simulink model "simulation_model"  (R2022a)
settings: Solver=VariableStepAuto  StartTime=0.0  StopTime=inf  FixedStep=0.02  MaxStep=0.1  RelTol=1e-3
values from neighbouring files (symbols this model uses):
  psi0 = atan(yc/xc)    [close_example.m]    (also in example_m.m)
  xc = coordinate(1)    [close_example.m]    (also in example_m.m)
  yc = coordinate(2)    [close_example.m]    (also in example_m.m)
undefined symbols (not defined in the file or in its folder): fuel_rate, gamma_pb, Pose, sigbuilder_block
libraries: simulink_extras x4, robotlib x3, simulink x1
(part 3 of 3)

== matlab function simulation_model/Parameters of rocket 9M723 and atmosphere model/Aerodynamic characteristics 9M723 ==
  data: Ma input; C_X0 output; C_Xa2 output; x_sm input; C_Na_kadl output; C_Na_ster output; x_sp output; C_ma output; C_mq output; x_sp_kadl output; x_sp_ster output
%% function which calculates Aerodynamic Force and Moment Coefficients
% 
% Inputs:
% Ma - number of Mach;
% x_sm - coordinate center of gravity [m]
%
% Outputs:
% C_X0 - Axial force coefficient (\alpha_t = 0)
% C_Xa2 - Derivative of axial force coefficient after sin^2\alpha_t
% C_Na_kadl - Derivative of normal force coefficient after sin\alpha for monocoque
% C_Na_ster - Derivative of normal force coefficient after sin\alpha for fins
% x_sp - coordinate center of pressure [m]
% C_ma - Derivative after pitch moment coefficient slope after sin\alpha
% C_mq - Pitch damping coefficient
% x_sp_kadl - coordinate center of pressure for monocoque [m]
% x_sp_ster - coordinate center of pressure for fins [m]


function [C_X0, C_Xa2, C_Na_kadl, C_Na_ster, x_sp, C_ma, C_mq, x_sp_kadl, x_sp_ster] = fcn(Ma, x_sm)

% Center of Gravity
CG = [2.8 3 3.3 3.5 3.7 4 4.4];

% Aerodynamic_Force_Coefficients
% [     Mach      CX0     CX2     CX4     CNa    CNa3    CPN     CYpa   CXfore  CXbase    CNq ]
AFC = [  0.01   0.216    2.81    3.12    3.92    3.12    3.92    0.00   0.000   0.068   0.148
         0.40   0.217    2.81    3.25    4.05    3.25    4.05    0.00   0.000   0.062   0.155
         0.60   0.217    2.81    3.31    4.12    3.31    4.12    0.00   0.000   0.058   0.158
         0.70   0.218    3.05    3.34    4.12    3.34    4.12    0.00   0.000   0.056   0.163
         0.75   0.219    3.17    3.35    4.12    3.35    4.12    0.00   0.000   0.054   0.165
         0.80   0.220    3.29    3.36    4.12    3.36    4.12    0.00   0.000   0.053   0.168
         0.85   0.232    3.53    3.41    4.15    3.41    4.15    0.00   0.000   0.062   0.170
         0.88   0.237    3.65    3.43    4.16    3.43    4.16    0.00   0.000   0.066   0.171
         0.90   0.243    3.76    3.45    4.17    3.45    4.17    0.00   0.000   0.071   0.172
         0.93   0.263    4.01    3.48    4.18    3.48    4.18    0.00   0.000   0.090   0.173
         0.95   0.283    4.25    3.50    4.18    3.50    4.18    0.00   0.000   0.108   0.174
         0.98   0.304    4.54    3.53    4.20    3.53    4.20    0.00   0.000   0.108   0.196
         1.00   0.325    4.83    3.56    4.22    3.56    4.22    0.00   0.000   0.108   0.217
         1.02   0.322    5.12    3.57    4.25    3.57    4.25    0.00   0.000   0.107   0.215
         1.05   0.319    5.41    3.58    4.28    3.58    4.28    0.00   0.000   0.105   0.214
         1.10   0.318    6.00    3.60    4.28    3.60    4.28    0.00   0.000   0.104   0.214
         1.20   0.310    6.65    3.62    4.23    3.62    4.23    0.00   0.000   0.100   0.210
         1.35   0.302    6.07    3.65    4.15    3.65    4.15    0.00   0.000   0.098   0.203
         1.50   0.288    5.46    3.71    4.04    3.71    4.04    0.00   0.000   0.092   0.196
         1.75   0.264    4.84    3.82    3.97    3.82    3.97    0.00   0.000   0.082   0.182
         2.00   0.245    4.24    3.81    3.89    3.81    3.89    0.00   0.000   0.078   0.167
         2.25   0.226    3.94    3.78    3.81    3.78    3.81    0.00   0.000   0.073   0.153
         2.50   0.206    3.63    3.75    3.74    3.75    3.74    0.00   0.000   0.068   0.138
         3.00   0.179    3.08    3.60    3.66    3.60    3.66    0.00   0.000   0.068   0.112
         3.50   0.163    2.82    3.46    3.56    3.46    3.56    0.00   0.000   0.070   0.093
         4.00   0.147    2.57    3.32    3.45    3.32    3.45    0.00   0.000   0.073   0.074
         4.50   0.137    2.32    3.24    3.41    3.24    3.41    0.00   0.000   0.075   0.062
         5.00   0.128    2.07    3.15    3.37    3.15    3.37    0.00   0.000   0.077   0.051
         6.00   0.114    1.85    3.08    3.32    3.08    3.32    0.00   0.000   0.078   0.037
         8.00   0.106    1.76    3.04    3.32    3.04    3.32    0.00   0.000   0.085   0.021];

%Aerodynamic Moment Coefficients for CG = 2800 mm
%          [ Mach     Cma     Cma3    Cma5    Cmq     Cmq2   Cnpa@1  Cnpa@3   Cnpa@5    Clp     Cld]
AMC_2800 = [  0.01   -2.75   -2.75  -135.7  -135.7   0.00   0.00   0.00   0.00   0.000  -0.501  0.0039
         0.40   -3.28   -3.28  -140.5  -140.5   0.00   0.00   0.00   0.00   0.000  -0.564  0.0045
         0.60   -3.56   -3.56  -143.0  -143.0   0.00   0.00   0.00   0.00   0.000  -0.596  0.0048
         0.70   -3.59   -3.59  -143.5  -143.5   0.00   0.00   0.00   0.00   0.000  -0.602  0.0048
         0.75   -3.61   -3.61  -143.8  -143.8   0.00   0.00   0.00   0.00   0.000  -0.605  0.0048
         0.80   -3.62   -3.62  -144.0  -144.0   0.00   0.00   0.00   0.00   0.000  -0.608  0.0049
         0.85   -3.75   -3.75  -146.6  -146.6   0.00   0.00   0.00   0.00   0.000  -0.624  0.0050
         0.88   -3.82   -3.82  -147.9  -147.9   0.00   0.00   0.00   0.00   0.000  -0.633  0.0051
         0.90   -3.89   -3.89  -149.2  -149.2   0.00   0.00   0.00   0.00   0.000  -0.641  0.0052
         0.93   -3.94   -3.94  -151.1  -151.1   0.00   0.00   0.00   0.00   0.000  -0.649  0.0052
         0.95   -3.99   -3.99  -153.0  -153.0   0.00   0.00   0.00   0.00   0.000  -0.657  0.0053
         0.98   -4.08   -4.08  -155.8  -155.8   0.00   0.00   0.00   0.00   0.000  -0.664  0.0054
         1.00   -4.17   -4.17  -158.6  -158.6   0.00   0.00   0.00   0.00   0.000  -0.670  0.0055
         1.02   -4.31   -4.31  -159.0  -159.0   0.00   0.00   0.00   0.00   0.000  -0.671  0.0055
         1.05   -4.45   -4.45  -159.4  -159.4   0.00   0.00   0.00   0.00   0.000  -0.671  0.0055
         1.10   -4.47   -4.47  -163.7  -163.7   0.00   0.00   0.00   0.00   0.000  -0.672  0.0055
         1.20   -4.29   -4.29  -165.6  -165.6   0.00   0.00   0.00   0.00   0.000  -0.651  0.0053
         1.35   -4.06   -4.06  -167.1  -167.1   0.00   0.00   0.00   0.00   0.000  -0.623  0.0051
         1.50   -3.69   -3.69  -168.6  -168.6   0.00   0.00   0.00   0.00   0.000  -0.596  0.0048
         1.75   -3.55   -3.55  -171.8  -171.8   0.00   0.00   0.00   0.00   0.000  -0.587  0.0048
         2.00   -3.21   -3.21  -171.4  -171.4   0.00   0.00   0.00   0.00   0.000  -0.531  0.0043
         2.25   -2.91   -2.91  -170.1  -170.1   0.00   0.00   0.00   0.00   0.000  -0.492  0.0040
         2.50   -2.61   -2.61  -168.7  -168.7   0.00   0.00   0.00   0.00   0.000  -0.452  0.0036
         3.00   -2.23   -2.23  -164.4  -164.4   0.00   0.00   0.00   0.00   0.000  -0.399  0.0032
         3.50   -1.79   -1.79  -158.7  -158.7   0.00   0.00   0.00   0.00   0.000  -0.353  0.0028
         4.00   -1.35   -1.35  -153.0  -153.0   0.00   0.00   0.00   0.00   0.000  -0.307  0.0024
         4.50   -1.19   -1.19  -148.9  -148.9   0.00   0.00   0.00   0.00   0.000  -0.291  0.0022
         5.00   -1.02   -1.02  -144.7  -144.7   0.00   0.00   0.00   0.00   0.000  -0.275  0.0021
         6.00   -0.87   -0.87  -141.6  -141.6   0.00   0.00   0.00   0.00   0.000  -0.261  0.0020
         8.00   -0.83   -0.83  -140.4  -140.4   0.00   0.00   0.00   0.00   0.000  -0.257  0.0019];

%Aerodynamic Moment Coefficients for CG = 3000 mm
%          [ Mach     Cma     Cma3    Cma5    Cmq     Cmq2   Cnpa@1  Cnpa@3   Cnpa@5    Clp     Cld]
AMC_3000 = [0.01   -2.07   -2.07  -124.4  -124.4   0.00   0.00   0.00   0.00   0.000  -0.501  0.0039
         0.40   -2.58   -2.58  -128.8  -128.8   0.00   0.00   0.00   0.00   0.000  -0.564  0.0045
         0.60   -2.84   -2.84  -131.1  -131.1   0.00   0.00   0.00   0.00   0.000  -0.596  0.0048
         0.70   -2.87   -2.87  -131.5  -131.5   0.00   0.00   0.00   0.00   0.000  -0.602  0.0048
         0.75   -2.88   -2.88  -131.7  -131.7   0.00   0.00   0.00   0.00   0.000  -0.605  0.0048
         0.80   -2.89   -2.89  -132.0  -132.0   0.00   0.00   0.00   0.00   0.000  -0.608  0.0049
         0.85   -3.01   -3.01  -134.5  -134.5   0.00   0.00   0.00   0.00   0.000  -0.624  0.0050
         0.88   -3.08   -3.08  -135.8  -135.8   0.00   0.00   0.00   0.00   0.000  -0.633  0.0051
         0.90   -3.14   -3.14  -137.1  -137.1   0.00   0.00   0.00   0.00   0.000  -0.641  0.0052
         0.93   -3.18   -3.18  -138.9  -138.9   0.00   0.00   0.00   0.00   0.000  -0.649  0.0052
         0.95   -3.23   -3.23  -140.7  -140.7   0.00   0.00   0.00   0.00   0.000  -0.657  0.0053
         0.98   -3.32   -3.32  -143.5  -143.5   0.00   0.00   0.00   0.00   0.000  -0.664  0.0054
         1.00   -3.40   -3.40  -146.2  -146.2   0.00   0.00   0.00   0.00   0.000  -0.670  0.0055
         1.02   -3.53   -3.53  -146.6  -146.6   0.00   0.00   0.00   0.00   0.000  -0.671  0.0055
         1.05   -3.67   -3.67  -147.0  -147.0   0.00   0.00   0.00   0.00   0.000  -0.671  0.0055
         1.10   -3.68   -3.68  -151.4  -151.4   0.00   0.00   0.00   0.00   0.000  -0.672  0.0055
         1.20   -3.51   -3.51  -153.6  -153.6   0.00   0.00   0.00   0.00   0.000  -0.651  0.0053
         1.35   -3.26   -3.26  -155.8  -155.8   0.00   0.00   0.00   0.00   0.000  -0.623  0.0051
         1.50   -2.88   -2.88  -158.5  -158.5   0.00   0.00   0.00   0.00   0.000  -0.596  0.0048
         1.75   -2.72   -2.72  -161.8  -161.8   0.00   0.00   0.00   0.00   0.000  -0.587  0.0048
         2.00   -2.38   -2.38  -161.7  -161.7   0.00   0.00   0.00   0.00   0.000  -0.531  0.0043
         2.25   -2.08   -2.08  -160.7  -160.7   0.00   0.00   0.00   0.00   0.000  -0.492  0.0040
         2.50   -1.79   -1.79  -159.7  -159.7   0.00   0.00   0.00   0.00   0.000  -0.452  0.0036
         3.00   -1.45   -1.45  -155.8  -155.8   0.00   0.00   0.00   0.00   0.000  -0.399  0.0032
         3.50   -1.04   -1.04  -150.5  -150.5   0.00   0.00   0.00   0.00   0.000  -0.353  0.0028
         4.00   -0.63   -0.63  -145.1  -145.1   0.00   0.00   0.00   0.00   0.000  -0.307  0.0024
         4.50   -0.48   -0.48  -141.1  -141.1   0.00   0.00   0.00   0.00   0.000  -0.291  0.0022
         5.00   -0.33   -0.33  -137.0  -137.0   0.00   0.00   0.00   0.00   0.000  -0.275  0.0021
         6.00   -0.20   -0.20  -134.1  -134.1   0.00   0.00   0.00   0.00   0.000  -0.261  0.0020
         8.00   -0.17   -0.17  -132.9  -132.9   0.00   0.00   0.00   0.00   0.000  -0.257  0.0019];

%Aerodynamic Moment Coefficients for CG = 3300 mm
%         [ Mach     Cma     Cma3    Cma5    Cmq     Cmq2   Cnpa@1  Cnpa@3   Cnpa@5    Clp     Cld]
AMC_3300 = [0.01   -1.05   -1.05  -107.9  -107.9   0.00   0.00   0.00   0.00   0.000  -0.501  0.0039
         0.40   -1.52   -1.52  -111.6  -111.6   0.00   0.00   0.00   0.00   0.000  -0.564  0.0045
         0.60   -1.76   -1.76  -113.5  -113.5   0.00   0.00   0.00   0.00   0.000  -0.596  0.0048
         0.70   -1.78   -1.78  -113.9  -113.9   0.00   0.00   0.00   0.00   0.000  -0.602  0.0048
         0.75   -1.79   -1.79  -114.1  -114.1   0.00   0.00   0.00   0.00   0.000  -0.605  0.0048
         0.80   -1.80   -1.80  -114.3  -114.3   0.00   0.00   0.00   0.00   0.000  -0.608  0.0049
         0.85   -1.90   -1.90  -116.8  -116.8   0.00   0.00   0.00   0.00   0.000  -0.624  0.0050
         0.88   -1.96   -1.96  -118.0  -118.0   0.00   0.00   0.00   0.00   0.000  -0.633  0.0051
         0.90   -2.01   -2.01  -119.2  -119.2   0.00   0.00   0.00   0.00   0.000  -0.641  0.0052
         0.93   -2.05   -2.05  -121.0  -121.0   0.00   0.00   0.00   0.00   0.000  -0.649  0.0052
         0.95   -2.09   -2.09  -122.7  -122.7   0.00   0.00   0.00   0.00   0.000  -0.657  0.0053
         0.98   -2.16   -2.16  -125.4  -125.4   0.00   0.00   0.00   0.00   0.000  -0.664  0.0054
         1.00   -2.24   -2.24  -128.0  -128.0   0.00   0.00   0.00   0.00   0.000  -0.670  0.0055
         1.02   -2.37   -2.37  -128.4  -128.4   0.00   0.00   0.00   0.00   0.000  -0.671  0.0055
         1.05   -2.50   -2.50  -128.8  -128.8   0.00   0.00   0.00   0.00   0.000  -0.671  0.0055
         1.10   -2.51   -2.51  -133.3  -133.3   0.00   0.00   0.00   0.00   0.000  -0.672  0.0055
         1.20   -2.33   -2.33  -135.9  -135.9   0.00   0.00   0.00   0.00   0.000  -0.651  0.0053
         1.35   -2.07   -2.07  -139.2  -139.2   0.00   0.00   0.00   0.00   0.000  -0.623  0.0051
         1.50   -1.67   -1.67  -143.8  -143.8   0.00   0.00   0.00   0.00   0.000  -0.596  0.0048
         1.75   -1.47   -1.47  -147.1  -147.1   0.00   0.00   0.00   0.00   0.000  -0.587  0.0048
         2.00   -1.14   -1.14  -147.6  -147.6   0.00   0.00   0.00   0.00   0.000  -0.531  0.0043
         2.25   -0.85   -0.85  -147.0  -147.0   0.00   0.00   0.00   0.00   0.000  -0.492  0.0040
         2.50   -0.57   -0.57  -146.5  -146.5   0.00   0.00   0.00   0.00   0.000  -0.452  0.0036
         3.00   -0.27   -0.27  -143.1  -143.1   0.00   0.00   0.00   0.00   0.000  -0.399  0.0032
         3.50    0.09    0.09  -138.3  -138.3   0.00   0.00   0.00   0.00   0.000  -0.353  0.0028
         4.00    0.45    0.45  -133.4  -133.4   0.00   0.00   0.00   0.00   0.000  -0.307  0.0024
         4.50    0.57    0.57  -129.5  -129.5   0.00   0.00   0.00   0.00   0.000  -0.291  0.0022
         5.00    0.69    0.69  -125.6  -125.6   0.00   0.00   0.00   0.00   0.000  -0.275  0.0021
         6.00    0.81    0.81  -122.9  -122.9   0.00   0.00   0.00   0.00   0.000  -0.261  0.0020
         8.00    0.83    0.83  -121.7  -121.7   0.00   0.00   0.00   0.00   0.000  -0.257  0.0019];

%Aerodynamic Moment Coefficients for CG = 3500 mm
%         [ Mach     Cma     Cma3    Cma5    Cmq     Cmq2   Cnpa@1  Cnpa@3   Cnpa@5    Clp     Cld]
AMC_3500 = [0.01   -0.37   -0.37   -97.1   -97.1   0.00   0.00   0.00   0.00   0.000  -0.501  0.0039
         0.40   -0.81   -0.81  -100.4  -100.4   0.00   0.00   0.00   0.00   0.000  -0.564  0.0045
         0.60   -1.04   -1.04  -102.1  -102.1   0.00   0.00   0.00   0.00   0.000  -0.596  0.0048
         0.70   -1.05   -1.05  -102.4  -102.4   0.00   0.00   0.00   0.00   0.000  -0.602  0.0048
         0.75   -1.06   -1.06  -102.6  -102.6   0.00   0.00   0.00   0.00   0.000  -0.605  0.0048
         0.80   -1.07   -1.07  -102.8  -102.8   0.00   0.00   0.00   0.00   0.000  -0.608  0.0049
         0.85   -1.16   -1.16  -105.2  -105.2   0.00   0.00   0.00   0.00   0.000  -0.624  0.0050
         0.88   -1.21   -1.21  -106.4  -106.4   0.00   0.00   0.00   0.00   0.000  -0.633  0.0051
         0.90   -1.26   -1.26  -107.6  -107.6   0.00   0.00   0.00   0.00   0.000  -0.641  0.0052
         0.93   -1.30   -1.30  -109.3  -109.3   0.00   0.00   0.00   0.00   0.000  -0.649  0.0052
         0.95   -1.33   -1.33  -111.0  -111.0   0.00   0.00   0.00   0.00   0.000  -0.657  0.0053
         0.98   -1.40   -1.40  -113.6  -113.6   0.00   0.00   0.00   0.00   0.000  -0.664  0.0054
         1.00   -1.46   -1.46  -116.2  -116.2   0.00   0.00   0.00   0.00   0.000  -0.670  0.0055
         1.02   -1.59   -1.59  -116.6  -116.6   0.00   0.00   0.00   0.00   0.000  -0.671  0.0055
         1.05   -1.72   -1.72  -117.0  -117.0   0.00   0.00   0.00   0.00   0.000  -0.671  0.0055
         1.10   -1.73   -1.73  -121.5  -121.5   0.00   0.00   0.00   0.00   0.000  -0.672  0.0055
         1.20   -1.54   -1.54  -124.5  -124.5   0.00   0.00   0.00   0.00   0.000  -0.651  0.0053
         1.35   -1.28   -1.28  -128.5  -128.5   0.00   0.00   0.00   0.00   0.000  -0.623  0.0051
         1.50   -0.86   -0.86  -134.2  -134.2   0.00   0.00   0.00   0.00   0.000  -0.596  0.0048
         1.75   -0.64   -0.64  -137.6  -137.6   0.00   0.00   0.00   0.00   0.000  -0.587  0.0048
         2.00   -0.31   -0.31  -138.5  -138.5   0.00   0.00   0.00   0.00   0.000  -0.531  0.0043
         2.25   -0.03   -0.03  -138.1  -138.1   0.00   0.00   0.00   0.00   0.000  -0.492  0.0040
         2.50    0.25    0.25  -137.8  -137.8   0.00   0.00   0.00   0.00   0.000  -0.452  0.0036
         3.00    0.51    0.51  -134.8  -134.8   0.00   0.00   0.00   0.00   0.000  -0.399  0.0032
         3.50    0.84    0.84  -130.3  -130.3   0.00   0.00   0.00   0.00   0.000  -0.353  0.0028
         4.00    1.17    1.17  -125.8  -125.8   0.00   0.00   0.00   0.00   0.000  -0.307  0.0024
         4.50    1.28    1.28  -122.0  -122.0   0.00   0.00   0.00   0.00   0.000  -0.291  0.0022
         5.00    1.38    1.38  -118.2  -118.2   0.00   0.00   0.00   0.00   0.000  -0.275  0.0021
         6.00    1.48    1.48  -115.5  -115.5   0.00   0.00   0.00   0.00   0.000  -0.261  0.0020
         8.00    1.49    1.49  -114.4  -114.4   0.00   0.00   0.00   0.00   0.000  -0.257  0.0019];

%Aerodynamic Moment Coefficients for CG = 3700 mm
%          [ Mach     Cma     Cma3    Cma5    Cmq     Cmq2   Cnpa@1  Cnpa@3   Cnpa@5    Clp     Cld]
AMC_3700 = [0.01    0.31    0.31   -86.4   -86.4   0.00   0.00   0.00   0.00   0.000  -0.501  0.0039
         0.40   -0.11   -0.11   -89.4   -89.4   0.00   0.00   0.00   0.00   0.000  -0.564  0.0045
         0.60   -0.32   -0.32   -90.9   -90.9   0.00   0.00   0.00   0.00   0.000  -0.596  0.0048
         0.70   -0.33   -0.33   -91.2   -91.2   0.00   0.00   0.00   0.00   0.000  -0.602  0.0048
         0.75   -0.33   -0.33   -91.3   -91.3   0.00   0.00   0.00   0.00   0.000  -0.605  0.0048
         0.80   -0.34   -0.34   -91.5   -91.5   0.00   0.00   0.00   0.00   0.000  -0.608  0.0049
         0.85   -0.42   -0.42   -93.8   -93.8   0.00   0.00   0.00   0.00   0.000  -0.624  0.0050
         0.88   -0.47   -0.47   -95.0   -95.0   0.00   0.00   0.00   0.00   0.000  -0.633  0.0051
         0.90   -0.51   -0.51   -96.2   -96.2   0.00   0.00   0.00   0.00   0.000  -0.641  0.0052
         0.93   -0.54   -0.54   -97.9   -97.9   0.00   0.00   0.00   0.00   0.000  -0.649  0.0052
         0.95   -0.57   -0.57   -99.5   -99.5   0.00   0.00   0.00   0.00   0.000  -0.657  0.0053
         0.98   -0.63   -0.63  -102.1  -102.1   0.00   0.00   0.00   0.00   0.000  -0.664  0.0054
         1.00   -0.69   -0.69  -104.7  -104.7   0.00   0.00   0.00   0.00   0.000  -0.670  0.0055
         1.02   -0.82   -0.82  -105.1  -105.1   0.00   0.00   0.00   0.00   0.000  -0.671  0.0055
         1.05   -0.94   -0.94  -105.4  -105.4   0.00   0.00   0.00   0.00   0.000  -0.671  0.0055
         1.10   -0.94   -0.94  -109.9  -109.9   0.00   0.00   0.00   0.00   0.000  -0.672  0.0055
         1.20   -0.75   -0.75  -113.2  -113.2   0.00   0.00   0.00   0.00   0.000  -0.651  0.0053
         1.35   -0.48   -0.48  -118.0  -118.0   0.00   0.00   0.00   0.00   0.000  -0.623  0.0051
         1.50   -0.06   -0.06  -124.8  -124.8   0.00   0.00   0.00   0.00   0.000  -0.596  0.0048
         1.75    0.19    0.19  -128.3  -128.3   0.00   0.00   0.00   0.00   0.000  -0.587  0.0048
         2.00    0.52    0.52  -129.5  -129.5   0.00   0.00   0.00   0.00   0.000  -0.531  0.0043
         2.25    0.79    0.79  -129.4  -129.4   0.00   0.00   0.00   0.00   0.000  -0.492  0.0040
         2.50    1.07    1.07  -129.3  -129.3   0.00   0.00   0.00   0.00   0.000  -0.452  0.0036
         3.00    1.29    1.29  -126.7  -126.7   0.00   0.00   0.00   0.00   0.000  -0.399  0.0032
         3.50    1.60    1.60  -122.4  -122.4   0.00   0.00   0.00   0.00   0.000  -0.353  0.0028
         4.00    1.89    1.89  -118.2  -118.2   0.00   0.00   0.00   0.00   0.000  -0.307  0.0024
         4.50    1.98    1.98  -114.5  -114.5   0.00   0.00   0.00   0.00   0.000  -0.291  0.0022
         5.00    2.07    2.07  -110.8  -110.8   0.00   0.00   0.00   0.00   0.000  -0.275  0.0021
         6.00    2.14    2.14  -108.2  -108.2   0.00   0.00   0.00   0.00   0.000  -0.261  0.0020
         8.00    2.15    2.15  -107.1  -107.1   0.00   0.00   0.00   0.00   0.000  -0.257  0.0019];

%Aerodynamic Moment Coefficients for CG = 4000 mm
%         [ Mach     Cma     Cma3    Cma5    Cmq     Cmq2   Cnpa@1  Cnpa@3   Cnpa@5    Clp     Cld]
AMC_4000 = [0.01    1.32    1.32   -70.8   -70.8   0.00   0.00   0.00   0.00   0.000  -0.501  0.0039
         0.40    0.95    0.95   -73.2   -73.2   0.00   0.00   0.00   0.00   0.000  -0.564  0.0045
         0.60    0.76    0.76   -74.4   -74.4   0.00   0.00   0.00   0.00   0.000  -0.596  0.0048
         0.70    0.76    0.76   -74.7   -74.7   0.00   0.00   0.00   0.00   0.000  -0.602  0.0048
         0.75    0.76    0.76   -74.8   -74.8   0.00   0.00   0.00   0.00   0.000  -0.605  0.0048
         0.80    0.76    0.76   -74.9   -74.9   0.00   0.00   0.00   0.00   0.000  -0.608  0.0049
         0.85    0.69    0.69   -77.2   -77.2   0.00   0.00   0.00   0.00   0.000  -0.624  0.0050
         0.88    0.65    0.65   -78.3   -78.3   0.00   0.00   0.00   0.00   0.000  -0.633  0.0051
         0.90    0.61    0.61   -79.5   -79.5   0.00   0.00   0.00   0.00   0.000  -0.641  0.0052
         0.93    0.59    0.59   -81.1   -81.1   0.00   0.00   0.00   0.00   0.000  -0.649  0.0052
         0.95    0.57    0.57   -82.8   -82.8   0.00   0.00   0.00   0.00   0.000  -0.657  0.0053
         0.98    0.52    0.52   -85.3   -85.3   0.00   0.00   0.00   0.00   0.000  -0.664  0.0054
         1.00    0.47    0.47   -87.8   -87.8   0.00   0.00   0.00   0.00   0.000  -0.670  0.0055
         1.02    0.35    0.35   -88.1   -88.1   0.00   0.00   0.00   0.00   0.000  -0.671  0.0055
         1.05    0.23    0.23   -88.5   -88.5   0.00   0.00   0.00   0.00   0.000  -0.671  0.0055
         1.10    0.23    0.23   -93.1   -93.1   0.00   0.00   0.00   0.00   0.000  -0.672  0.0055
         1.20    0.43    0.43   -96.8   -96.8   0.00   0.00   0.00   0.00   0.000  -0.651  0.0053
         1.35    0.71    0.71  -102.6  -102.6   0.00   0.00   0.00   0.00   0.000  -0.623  0.0051
         1.50    1.15    1.15  -111.2  -111.2   0.00   0.00   0.00   0.00   0.000  -0.596  0.0048
         1.75    1.43    1.43  -114.7  -114.7   0.00   0.00   0.00   0.00   0.000  -0.587  0.0048
         2.00    1.76    1.76  -116.4  -116.4   0.00   0.00   0.00   0.00   0.000  -0.531  0.0043
         2.25    2.03    2.03  -116.6  -116.6   0.00   0.00   0.00   0.00   0.000  -0.492  0.0040
         2.50    2.29    2.29  -116.9  -116.9   0.00   0.00   0.00   0.00   0.000  -0.452  0.0036
         3.00    2.47    2.47  -114.7  -114.7   0.00   0.00   0.00   0.00   0.000  -0.399  0.0032
         3.50    2.72    2.72  -110.9  -110.9   0.00   0.00   0.00   0.00   0.000  -0.353  0.0028
         4.00    2.98    2.98  -107.0  -107.0   0.00   0.00   0.00   0.00   0.000  -0.307  0.0024
         4.50    3.04    3.04  -103.5  -103.5   0.00   0.00   0.00   0.00   0.000  -0.291  0.0022
         5.00    3.09    3.09  -100.0  -100.0   0.00   0.00   0.00   0.00   0.000  -0.275  0.0021
         6.00    3.15    3.15   -97.5   -97.5   0.00   0.00   0.00   0.00   0.000  -0.261  0.0020
         8.00    3.14    3.14   -96.4   -96.4   0.00   0.00   0.00   0.00   0.000  -0.257  0.0019];

%Aerodynamic Moment Coefficients for CG = 4400 mm
%          [ Mach     Cma     Cma3    Cma5    Cmq     Cmq2   Cnpa@1  Cnpa@3   Cnpa@5    Clp     Cld]
AMC_4400 = [0.01    2.68    2.68   -50.5   -50.5   0.00   0.00   0.00   0.00   0.000  -0.501  0.0039
         0.40    2.36    2.36   -52.3   -52.3   0.00   0.00   0.00   0.00   0.000  -0.564  0.0045
         0.60    2.20    2.20   -53.2   -53.2   0.00   0.00   0.00   0.00   0.000  -0.596  0.0048
         0.70    2.21    2.21   -53.4   -53.4   0.00   0.00   0.00   0.00   0.000  -0.602  0.0048
         0.75    2.22    2.22   -53.5   -53.5   0.00   0.00   0.00   0.00   0.000  -0.605  0.0048
         0.80    2.22    2.22   -53.6   -53.6   0.00   0.00   0.00   0.00   0.000  -0.608  0.0049
         0.85    2.17    2.17   -55.8   -55.8   0.00   0.00   0.00   0.00   0.000  -0.624  0.0050
         0.88    2.14    2.14   -56.9   -56.9   0.00   0.00   0.00   0.00   0.000  -0.633  0.0051
         0.90    2.11    2.11   -58.0   -58.0   0.00   0.00   0.00   0.00   0.000  -0.641  0.0052
         0.93    2.10    2.10   -59.6   -59.6   0.00   0.00   0.00   0.00   0.000  -0.649  0.0052
         0.95    2.09    2.09   -61.2   -61.2   0.00   0.00   0.00   0.00   0.000  -0.657  0.0053
         0.98    2.05    2.05   -63.6   -63.6   0.00   0.00   0.00   0.00   0.000  -0.664  0.0054
         1.00    2.01    2.01   -66.0   -66.0   0.00   0.00   0.00   0.00   0.000  -0.670  0.0055
         1.02    1.90    1.90   -66.4   -66.4   0.00   0.00   0.00   0.00   0.000  -0.671  0.0055
         1.05    1.78    1.78   -66.8   -66.8   0.00   0.00   0.00   0.00   0.000  -0.671  0.0055
         1.10    1.80    1.80   -71.4   -71.4   0.00   0.00   0.00   0.00   0.000  -0.672  0.0055
         1.20    2.00    2.00   -75.6   -75.6   0.00   0.00   0.00   0.00   0.000  -0.651  0.0053
         1.35    2.30    2.30   -82.8   -82.8   0.00   0.00   0.00   0.00   0.000  -0.623  0.0051
         1.50    2.77    2.77   -93.7   -93.7   0.00   0.00   0.00   0.00   0.000  -0.596  0.0048
         1.75    3.09    3.09   -97.3   -97.3   0.00   0.00   0.00   0.00   0.000  -0.587  0.0048
         2.00    3.42    3.42   -99.5   -99.5   0.00   0.00   0.00   0.00   0.000  -0.531  0.0043
         2.25    3.67    3.67  -100.2  -100.2   0.00   0.00   0.00   0.00   0.000  -0.492  0.0040
         2.50    3.92    3.92  -100.9  -100.9   0.00   0.00   0.00   0.00   0.000  -0.452  0.0036
         3.00    4.03    4.03   -99.2   -99.2   0.00   0.00   0.00   0.00   0.000  -0.399  0.0032
         3.50    4.23    4.23   -95.9   -95.9   0.00   0.00   0.00   0.00   0.000  -0.353  0.0028
         4.00    4.42    4.42   -92.5   -92.5   0.00   0.00   0.00   0.00   0.000  -0.307  0.0024
         4.50    4.44    4.44   -89.2   -89.2   0.00   0.00   0.00   0.00   0.000  -0.291  0.0022
         5.00    4.46    4.46   -85.8   -85.8   0.00   0.00   0.00   0.00   0.000  -0.275  0.0021
         6.00    4.49    4.49   -83.5   -83.5   0.00   0.00   0.00   0.00   0.000  -0.261  0.0020
         8.00    4.46    4.46   -82.4   -82.4   0.00   0.00   0.00   0.00   0.000  -0.257  0.0019];

% Fin Set Component Aerodynamic Coefficients
%          [ Mach   Cxbody   Cxgrv   Cxfin1  Cxfin2  Cxfin3   CNaB    CPNB   CNaF1   CPNF1   CNaF2   CPNF2   CNaF3   CPNF3]
FIN_2800 = [ 0.010   0.212   0.000   0.004   0.000   0.000    2.22    2.48    0.90    7.48    0.00    0.00    0.00    0.00
       0.400   0.212   0.000   0.004   0.000   0.000    2.22    2.47    1.03    7.48    0.00    0.00    0.00    0.00
       0.600   0.212   0.000   0.004   0.000   0.000    2.22    2.47    1.09    7.48    0.00    0.00    0.00    0.00
       0.700   0.213   0.000   0.005   0.000   0.000    2.23    2.46    1.10    7.47    0.00    0.00    0.00    0.00
       0.750   0.214   0.000   0.005   0.000   0.000    2.24    2.46    1.11    7.47    0.00    0.00    0.00    0.00
       0.800   0.215   0.000   0.006   0.000   0.000    2.24    2.45    1.12    7.47    0.00    0.00    0.00    0.00
       0.850   0.225   0.000   0.006   0.000   0.000    2.25    2.45    1.15    7.47    0.00    0.00    0.00    0.00
       0.875   0.230   0.000   0.007   0.000   0.000    2.26    2.44    1.17    7.47    0.00    0.00    0.00    0.00
       0.900   0.236   0.000   0.007   0.000   0.000    2.27    2.44    1.18    7.47    0.00    0.00    0.00    0.00
       0.925   0.255   0.000   0.007   0.000   0.000    2.27    2.44    1.20    7.47    0.00    0.00    0.00    0.00
       0.950   0.275   0.000   0.007   0.000   0.000    2.28    2.43    1.22    7.47    0.00    0.00    0.00    0.00
       0.975   0.296   0.000   0.008   0.000   0.000    2.29    2.44    1.23    7.47    0.00    0.00    0.00    0.00
       1.000   0.317   0.000   0.008   0.000   0.000    2.31    2.45    1.25    7.47    0.00    0.00    0.00    0.00
       1.025   0.314   0.000   0.008   0.000   0.000    2.32    2.50    1.25    7.50    0.00    0.00    0.00    0.00
       1.050   0.311   0.000   0.008   0.000   0.000    2.33    2.55    1.25    7.52    0.00    0.00    0.00    0.00
       1.100   0.310   0.000   0.008   0.000   0.000    2.35    2.53    1.26    7.56    0.00    0.00    0.00    0.00
       1.200   0.303   0.000   0.007   0.000   0.000    2.41    2.54    1.21    7.57    0.00    0.00    0.00    0.00
       1.350   0.294   0.000   0.007   0.000   0.000    2.49    2.56    1.16    7.58    0.00    0.00    0.00    0.00
       1.500   0.281   0.000   0.007   0.000   0.000    2.60    2.52    1.11    7.58    0.00    0.00    0.00    0.00
       1.750   0.258   0.000   0.007   0.000   0.000    2.72    2.52    1.09    7.58    0.00    0.00    0.00    0.00
       2.000   0.239   0.000   0.007   0.000   0.000    2.82    2.59    0.99    7.59    0.00    0.00    0.00    0.00
       2.250   0.219   0.000   0.007   0.000   0.000    2.87    2.62    0.91    7.59    0.00    0.00    0.00    0.00
       2.500   0.200   0.000   0.007   0.000   0.000    2.92    2.64    0.83    7.60    0.00    0.00    0.00    0.00
       3.000   0.173   0.000   0.006   0.000   0.000    2.88    2.67    0.72    7.60    0.00    0.00    0.00    0.00
       3.500   0.156   0.000   0.007   0.000   0.000    2.83    2.66    0.63    7.60    0.00    0.00    0.00    0.00
       4.000   0.140   0.000   0.007   0.000   0.000    2.78    2.64    0.54    7.60    0.00    0.00    0.00    0.00
       4.500   0.131   0.000   0.007   0.000   0.000    2.73    2.63    0.51    7.60    0.00    0.00    0.00    0.00
       5.000   0.121   0.000   0.006   0.000   0.000    2.68    2.61    0.48    7.61    0.00    0.00    0.00    0.00
       6.000   0.108   0.000   0.006   0.000   0.000    2.63    2.59    0.45    7.61    0.00    0.00    0.00    0.00
       8.000   0.100   0.000   0.006   0.000   0.000    2.60    2.58    0.44    7.61    0.00    0.00    0.00    0.00];

% calculate Aerodynamic Force and Moment Coefficients for Ma <= 0
if Ma <= 0
    C_X0 = AFC(1,2);
    C_Xa2 = AFC(1,3);
    C_Na_kadl = FIN_2800(1,7);
    C_Na_ster = FIN_2800(1,9);
    x_sp = AFC(1,7).*0.92;
    x_sp_kadl = FIN_2800(1,8).*0.92;
    x_sp_ster = FIN_2800(1,10).*0.92;
    
    % interpolation of C_ma
    C_ma2800 = AMC_2800(1,2);
    C_ma3000 = AMC_3000(1,2);
    C_ma3300 = AMC_3300(1,2);
    C_ma3500 = AMC_3500(1,2);
    C_ma3700 = AMC_3700(1,2);
    C_ma4000 = AMC_4000(1,2);
    C_ma4400 = AMC_4400(1,2);
    p = polyfit(CG,[C_ma2800 C_ma3000 C_ma3300 C_ma3500 C_ma3700 C_ma4000 C_ma4400],2);
    C_ma = polyval(p,x_sm);
    
    % interpolation of C_mq
    C_mq2800 = AMC_2800(1,4);
    C_mq3000 = AMC_3000(1,4);
    C_mq3300 = AMC_3300(1,4);
    C_mq3500 = AMC_3500(1,4);
    C_mq3700 = AMC_3700(1,4);
    C_mq4000 = AMC_4000(1,4);
    C_mq4400 = AMC_4400(1,4);
    p = polyfit(CG,[C_mq2800 C_mq3000 C_mq3300 C_mq3500 C_mq3700 C_mq4000 C_mq4400],2);
    C_mq = polyval(p,x_sm);
   
% calculate Aerodynamic Force and Moment Coefficients for Ma >= 8      
elseif Ma >= 8
    C_X0 = AFC(end,2);
    C_Xa2 = AFC(end,3);
    C_Na_kadl = FIN_2800(end,7);
    C_Na_ster = FIN_2800(end,9); 
    x_sp = AFC(end,7).*0.92;
    x_sp_kadl = FIN_2800(end,8).*0.92;
    x_sp_ster = FIN_2800(end,10).*0.92;
    
    % interpolation of C_ma
    C_ma2800 = AMC_2800(end,2);
    C_ma3000 = AMC_3000(end,2);
    C_ma3300 = AMC_3300(end,2);
    C_ma3500 = AMC_3500(end,2);
    C_ma3700 = AMC_3700(end,2);
    C_ma4000 = AMC_4000(end,2);
    C_ma4400 = AMC_4400(end,2);
    p = polyfit(CG,[C_ma2800 C_ma3000 C_ma3300 C_ma3500 C_ma3700 C_ma4000 C_ma4400],2);
    C_ma = polyval(p,x_sm);
    
    % interpolation of C_mq
    C_mq2800 = AMC_2800(end,4);
    C_mq3000 = AMC_3000(end,4);
    C_mq3300 = AMC_3300(end,4);
    C_mq3500 = AMC_3500(end,4);
    C_mq3700 = AMC_3700(end,4);
    C_mq4000 = AMC_4000(end,4);
    C_mq4400 = AMC_4400(end,4);
    p = polyfit(CG,[C_mq2800 C_mq3000 C_mq3300 C_mq3500 C_mq3700 C_mq4000 C_mq4400],2);
    C_mq = polyval(p,x_sm);

% calculate Aerodynamic Force and Moment Coefficients for Ma > 0 and Ma < 0.01
elseif Ma > 0 && Ma < AFC(1,1)
    C_X0 = AFC(1,2)/AFC(1,1)*Ma+(AFC(1,2)-AFC(1,2)/AFC(1,1)*AFC(1,1));
    C_Xa2 = AFC(1,3)/AFC(1,1)*Ma+(AFC(1,3)-AFC(1,3)/AFC(1,1)*AFC(1,1));
    C_Na_kadl = FIN_2800(1,7)/AFC(1,1)*Ma+(FIN_2800(1,7)-FIN_2800(1,7)/AFC(1,1)*AFC(1,1));
    C_Na_ster = FIN_2800(1,9)/AFC(1,1)*Ma+(FIN_2800(1,9)-FIN_2800(1,9)/AFC(1,1)*AFC(1,1));
    x_sp = AFC(1,7).*0.92/AFC(1,1)*Ma+(AFC(1,7).*0.92-AFC(1,7).*0.92/AFC(1,1)*AFC(1,1));
    x_sp_kadl = FIN_2800(1,8).*0.92/AFC(1,1)*Ma+(FIN_2800(1,8).*0.92-FIN_2800(1,8).*0.92/AFC(1,1)*AFC(1,1));
    x_sp_ster = FIN_2800(1,10).*0.92/AFC(1,1)*Ma+(FIN_2800(1,10).*0.92-FIN_2800(1,10).*0.92/AFC(1,1)*AFC(1,1));

    % interpolation of C_ma
    C_ma2800 = AMC_2800(1,2)/AFC(1,1)*Ma+(AMC_2800(1,2)-AMC_2800(1,2)/AFC(1,1)*AFC(1,1));
    C_ma3000 = AMC_3000(1,2)/AFC(1,1)*Ma+(AMC_3000(1,2)-AMC_3000(1,2)/AFC(1,1)*AFC(1,1));
    C_ma3300 = AMC_3300(1,2)/AFC(1,1)*Ma+(AMC_3300(1,2)-AMC_3300(1,2)/AFC(1,1)*AFC(1,1));
    C_ma3500 = AMC_3500(1,2)/AFC(1,1)*Ma+(AMC_3500(1,2)-AMC_3500(1,2)/AFC(1,1)*AFC(1,1));
    C_ma3700 = AMC_3700(1,2)/AFC(1,1)*Ma+(AMC_3700(1,2)-AMC_3700(1,2)/AFC(1,1)*AFC(1,1));
    C_ma4000 = AMC_4000(1,2)/AFC(1,1)*Ma+(AMC_4000(1,2)-AMC_4000(1,2)/AFC(1,1)*AFC(1,1));
    C_ma4400 = AMC_4400(1,2)/AFC(1,1)*Ma+(AMC_4400(1,2)-AMC_4400(1,2)/AFC(1,1)*AFC(1,1));
    p = polyfit(CG,[C_ma2800 C_ma3000 C_ma3300 C_ma3500 C_ma3700 C_ma4000 C_ma4400],2);
    C_ma = polyval(p,x_sm);
    
    % interpolation of C_mq
    C_mq2800 = AMC_2800(1,4)/AFC(1,1)*Ma+(AMC_2800(1,4)-AMC_2800(1,4)/AFC(1,1)*AFC(1,1));
    C_mq3000 = AMC_3000(1,4)/AFC(1,1)*Ma+(AMC_3000(1,4)-AMC_3000(1,4)/AFC(1,1)*AFC(1,1));
    C_mq3300 = AMC_3300(1,4)/AFC(1,1)*Ma+(AMC_3300(1,4)-AMC_3300(1,4)/AFC(1,1)*AFC(1,1));
    C_mq3500 = AMC_3500(1,4)/AFC(1,1)*Ma+(AMC_3500(1,4)-AMC_3500(1,4)/AFC(1,1)*AFC(1,1));
    C_mq3700 = AMC_3700(1,4)/AFC(1,1)*Ma+(AMC_3700(1,4)-AMC_3700(1,4)/AFC(1,1)*AFC(1,1));
    C_mq4000 = AMC_4000(1,4)/AFC(1,1)*Ma+(AMC_4000(1,4)-AMC_4000(1,4)/AFC(1,1)*AFC(1,1));
    C_mq4400 = AMC_4400(1,4)/AFC(1,1)*Ma+(AMC_4400(1,4)-AMC_4400(1,4)/AFC(1,1)*AFC(1,1));
    p = polyfit(CG,[C_mq2800 C_mq3000 C_mq3300 C_mq3500 C_mq3700 C_mq4000 C_mq4400],2);
    C_mq = polyval(p,x_sm);

% calculate Aerodynamic Force and Moment Coefficients for Ma > 0 and Ma < 8
else
    C_X0 = AFC(1,2)/AFC(1,1)*Ma+(AFC(1,2)-AFC(1,2)/AFC(1,1)*AFC(1,1));
    C_Xa2 = AFC(1,3)/AFC(1,1)*Ma+(AFC(1,3)-AFC(1,3)/AFC(1,1)*AFC(1,1));
    C_Na_kadl = FIN_2800(1,7)/AFC(1,1)*Ma+(FIN_2800(1,7)-FIN_2800(1,7)/AFC(1,1)*AFC(1,1));
    C_Na_ster = FIN_2800(1,9)/AFC(1,1)*Ma+(FIN_2800(1,9)-FIN_2800(1,9)/AFC(1,1)*AFC(1,1));
    x_sp = AFC(1,7).*0.92/AFC(1,1)*Ma+(AFC(1,7).*0.92-AFC(1,7).*0.92/AFC(1,1)*AFC(1,1));
    x_sp_kadl = FIN_2800(1,8).*0.92/AFC(1,1)*Ma+(FIN_2800(1,8).*0.92-FIN_2800(1,8).*0.92/AFC(1,1)*AFC(1,1));
    x_sp_ster = FIN_2800(1,10).*0.92/AFC(1,1)*Ma+(FIN_2800(1,10).*0.92-FIN_2800(1,10).*0.92/AFC(1,1)*AFC(1,1));

    % interpolation of C_ma
    C_ma2800 = AMC_2800(1,2)/AFC(1,1)*Ma+(AMC_2800(1,2)-AMC_2800(1,2)/AFC(1,1)*AFC(1,1));
    C_ma3000 = AMC_3000(1,2)/AFC(1,1)*Ma+(AMC_3000(1,2)-AMC_3000(1,2)/AFC(1,1)*AFC(1,1));
    C_ma3300 = AMC_3300(1,2)/AFC(1,1)*Ma+(AMC_3300(1,2)-AMC_3300(1,2)/AFC(1,1)*AFC(1,1));
    C_ma3500 = AMC_3500(1,2)/AFC(1,1)*Ma+(AMC_3500(1,2)-AMC_3500(1,2)/AFC(1,1)*AFC(1,1));
    C_ma3700 = AMC_3700(1,2)/AFC(1,1)*Ma+(AMC_3700(1,2)-AMC_3700(1,2)/AFC(1,1)*AFC(1,1));
    C_ma4000 = AMC_4000(1,2)/AFC(1,1)*Ma+(AMC_4000(1,2)-AMC_4000(1,2)/AFC(1,1)*AFC(1,1));
    C_ma4400 = AMC_4400(1,2)/AFC(1,1)*Ma+(AMC_4400(1,2)-AMC_4400(1,2)/AFC(1,1)*AFC(1,1));
    p = polyfit(CG,[C_ma2800 C_ma3000 C_ma3300 C_ma3500 C_ma3700 C_ma4000 C_ma4400],2);
    C_ma = polyval(p,x_sm);
    
    % interpolation of C_mq
    C_mq2800 = AMC_2800(1,4)/AFC(1,1)*Ma+(AMC_2800(1,4)-AMC_2800(1,4)/AFC(1,1)*AFC(1,1));
    C_mq3000 = AMC_3000(1,4)/AFC(1,1)*Ma+(AMC_3000(1,4)-AMC_3000(1,4)/AFC(1,1)*AFC(1,1));
    C_mq3300 = AMC_3300(1,4)/AFC(1,1)*Ma+(AMC_3300(1,4)-AMC_3300(1,4)/AFC(1,1)*AFC(1,1));
    C_mq3500 = AMC_3500(1,4)/AFC(1,1)*Ma+(AMC_3500(1,4)-AMC_3500(1,4)/AFC(1,1)*AFC(1,1));
    C_mq3700 = AMC_3700(1,4)/AFC(1,1)*Ma+(AMC_3700(1,4)-AMC_3700(1,4)/AFC(1,1)*AFC(1,1));
    C_mq4000 = AMC_4000(1,4)/AFC(1,1)*Ma+(AMC_4000(1,4)-AMC_4000(1,4)/AFC(1,1)*AFC(1,1));
    C_mq4400 = AMC_4400(1,4)/AFC(1,1)*Ma+(AMC_4400(1,4)-AMC_4400(1,4)/AFC(1,1)*AFC(1,1));
    p = polyfit(CG,[C_mq2800 C_mq3000 C_mq3300 C_mq3500 C_mq3700 C_mq4000 C_mq4400],2);
    C_mq = polyval(p,x_sm);
    
    % interpolation of Aerodynamic Coefficients
    i = 1;
    while Ma > AFC(i,1)
        C_X0 = (AFC(i,2)-AFC(i+1,2))/(AFC(i,1)-AFC(i+1,1))*Ma+(AFC(i,2)-(AFC(i,2)-AFC(i+1,2))/(AFC(i,1)-AFC(i+1,1))*AFC(i,1));
        C_Xa2 = (AFC(i,3)-AFC(i+1,3))/(AFC(i,1)-AFC(i+1,1))*Ma+(AFC(i,3)-(AFC(i,3)-AFC(i+1,3))/(AFC(i,1)-AFC(i+1,1))*AFC(i,1));
        C_Na_kadl = (FIN_2800(i,7)-FIN_2800(i+1,7))/(AFC(i,1)-AFC(i+1,1))*Ma+(FIN_2800(i,7)-(FIN_2800(i,7)-FIN_2800(i+1,7))/(AFC(i,1)-AFC(i+1,1))*AFC(i,1)); 
        C_Na_ster = (FIN_2800(i,9)-FIN_2800(i+1,9))/(AFC(i,1)-AFC(i+1,1))*Ma+(FIN_2800(i,9)-(FIN_2800(i,9)-FIN_2800(i+1,9))/(AFC(i,1)-AFC(i+1,1))*AFC(i,1));
        x_sp = (AFC(i,7).*0.92-AFC(i+1,7).*0.92)/(AFC(i,1)-AFC(i+1,1))*Ma+(AFC(i,7).*0.92-(AFC(i,7).*0.92-AFC(i+1,7).*0.92)/(AFC(i,1)-AFC(i+1,1))*AFC(i,1));
        x_sp_kadl = (FIN_2800(i,8).*0.92-FIN_2800(i+1,8).*0.92)/(AFC(i,1)-AFC(i+1,1))*Ma+(FIN_2800(i,8).*0.92-(FIN_2800(i,8).*0.92-FIN_2800(i+1,8).*0.92)/(AFC(i,1)-AFC(i+1,1))*AFC(i,1));
        x_sp_ster = (FIN_2800(i,10).*0.92-FIN_2800(i+1,10).*0.92)/(AFC(i,1)-AFC(i+1,1))*Ma+(FIN_2800(i,10).*0.92-(FIN_2800(i,10).*0.92-FIN_2800(i+1,10).*0.92)/(AFC(i,1)-AFC(i+1,1))*AFC(i,1));

        C_ma2800 = (AMC_2800(i,2)-AMC_2800(i+1,2))/(AFC(i,1)-AFC(i+1,1))*Ma+(AMC_2800(i,2)-(AMC_2800(i,2)-AMC_2800(i+1,2))/(AFC(i,1)-AFC(i+1,1))*AFC(i,1));
        C_ma3000 = (AMC_3000(i,2)-AMC_3000(i+1,2))/(AFC(i,1)-AFC(i+1,1))*Ma+(AMC_3000(i,2)-(AMC_3000(i,2)-AMC_3000(i+1,2))/(AFC(i,1)-AFC(i+1,1))*AFC(i,1));
        C_ma3300 = (AMC_3300(i,2)-AMC_3300(i+1,2))/(AFC(i,1)-AFC(i+1,1))*Ma+(AMC_3300(i,2)-(AMC_3300(i,2)-AMC_3300(i+1,2))/(AFC(i,1)-AFC(i+1,1))*AFC(i,1));
        C_ma3500 = (AMC_3500(i,2)-AMC_3500(i+1,2))/(AFC(i,1)-AFC(i+1,1))*Ma+(AMC_3500(i,2)-(AMC_3500(i,2)-AMC_3500(i+1,2))/(AFC(i,1)-AFC(i+1,1))*AFC(i,1));
        C_ma3700 = (AMC_3700(i,2)-AMC_3700(i+1,2))/(AFC(i,1)-AFC(i+1,1))*Ma+(AMC_3700(i,2)-(AMC_3700(i,2)-AMC_3700(i+1,2))/(AFC(i,1)-AFC(i+1,1))*AFC(i,1));
        C_ma4000 = (AMC_4000(i,2)-AMC_4000(i+1,2))/(AFC(i,1)-AFC(i+1,1))*Ma+(AMC_4000(i,2)-(AMC_4000(i,2)-AMC_4000(i+1,2))/(AFC(i,1)-AFC(i+1,1))*AFC(i,1));
        C_ma4400 = (AMC_4400(i,2)-AMC_4400(i+1,2))/(AFC(i,1)-AFC(i+1,1))*Ma+(AMC_4400(i,2)-(AMC_4400(i,2)-AMC_4400(i+1,2))/(AFC(i,1)-AFC(i+1,1))*AFC(i,1));
        p = polyfit(CG,[C_ma2800 C_ma3000 C_ma3300 C_ma3500 C_ma3700 C_ma4000 C_ma4400],2);
        C_ma = polyval(p,x_sm);
    
        C_mq2800 = (AMC_2800(i,4)-AMC_2800(i+1,4))/(AFC(i,1)-AFC(i+1,1))*Ma+(AMC_2800(i,4)-(AMC_2800(i,4)-AMC_2800(i+1,4))/(AFC(i,1)-AFC(i+1,1))*AFC(i,1));
        C_mq3000 = (AMC_3000(i,4)-AMC_3000(i+1,4))/(AFC(i,1)-AFC(i+1,1))*Ma+(AMC_3000(i,4)-(AMC_3000(i,4)-AMC_3000(i+1,4))/(AFC(i,1)-AFC(i+1,1))*AFC(i,1));
        C_mq3300 = (AMC_3300(i,4)-AMC_3300(i+1,4))/(AFC(i,1)-AFC(i+1,1))*Ma+(AMC_3300(i,4)-(AMC_3300(i,4)-AMC_3300(i+1,4))/(AFC(i,1)-AFC(i+1,1))*AFC(i,1));
        C_mq3500 = (AMC_3500(i,4)-AMC_3500(i+1,4))/(AFC(i,1)-AFC(i+1,1))*Ma+(AMC_3500(i,4)-(AMC_3500(i,4)-AMC_3500(i+1,4))/(AFC(i,1)-AFC(i+1,1))*AFC(i,1));
        C_mq3700 = (AMC_3700(i,4)-AMC_3700(i+1,4))/(AFC(i,1)-AFC(i+1,1))*Ma+(AMC_3700(i,4)-(AMC_3700(i,4)-AMC_3700(i+1,4))/(AFC(i,1)-AFC(i+1,1))*AFC(i,1));
        C_mq4000 = (AMC_4000(i,4)-AMC_4000(i+1,4))/(AFC(i,1)-AFC(i+1,1))*Ma+(AMC_4000(i,4)-(AMC_4000(i,4)-AMC_4000(i+1,4))/(AFC(i,1)-AFC(i+1,1))*AFC(i,1));
        C_mq4400 = (AMC_4400(i,4)-AMC_4400(i+1,4))/(AFC(i,1)-AFC(i+1,1))*Ma+(AMC_4400(i,4)-(AMC_4400(i,4)-AMC_4400(i+1,4))/(AFC(i,1)-AFC(i+1,1))*AFC(i,1));
        p = polyfit(CG,[C_mq2800 C_mq3000 C_mq3300 C_mq3500 C_mq3700 C_mq4000 C_mq4400],2);
        C_mq = polyval(p,x_sm);

        i = i + 1;
    end
end

== matlab function simulation_model/Missile dynamics model/Forces acting on the object /Gravity force ==
  data: m input; Q output; g input; phi input; theta input
%% function which calculates garvity force
% 
% Inputs:
% m - mass of rocket [kg]
% g - gravitational acceleration [m/s^2]
% phi - roll angle [rad]
% theta - pitch angle [rad]
%
% Outputs:
% Q - Gravity force [N]


function Q = fcn(m, g, phi, theta)

% calculate gravity force
Q = [-m*g*sin(theta); m*g*cos(theta)*sin(phi); m*g*cos(theta)*cos(phi)];

== matlab function simulation_model/Missile dynamics model/Forces acting on the object /Aerodynamic Force ==
  data: C_X0 input; R output; rho input; C_Na_ster input; C_Na_kadl input; alfa_t input; C_Xa2 input; U input; V input; W input; alfa input; beta input; delta_w input; delta_k input
%% function which calculates Components of the aerodynamic force
% 
% Inputs:
% C_X0 - Axial force coefficient (\alpha_t = 0)
% rho - air density [kg/m^3]
% C_Na_ster - Derivative of normal force coefficient after sin\alpha for fins
% C_Na_kadl - Derivative of normal force coefficient after sin\alpha for monocoque
% alfa_t - total angle of attack [rad]
% C_Xa2 - Derivative of axial force coefficient after sin^2\alpha_t
% U - velocity about x body axis [m/s]
% V - velocity about y body axis [m/s]
% W - velocity about z body axis [m/s]
% alfa - angle of attack [rad]
% beta - angle of sideslip [rad] 
% delta_w deflection of fins in axis Z [rad]
% delta_k - deflection of fins in axis Y [rad]
%
% Outputs:
% R - Aerodynamic force [N]


function R = fcn(C_X0, rho, C_Na_ster, C_Na_kadl, alfa_t, C_Xa2, U, V, W, alfa, beta, delta_w, delta_k)
R = zeros(3,1);

% calculate cross-sectional area
S = pi*(0.92/2)^2;

% calculate the absolute value of velocity
Vaer_bezwzgl = sqrt(U^2 + V^2 + W^2);

% calculate axial force
P_x = (C_X0 + C_Xa2*sin(alfa_t)^2)*0.5*rho*Vaer_bezwzgl^2*S;
P_x_x = -P_x;

% calculate normal force  and sideforce coefficients
C_N_y = C_Na_kadl*sin(beta) + C_Na_ster*sin(beta+delta_k);
C_N_z = C_Na_kadl*cos(beta)*sin(alfa) + C_Na_ster*cos(beta)*sin(alfa+delta_w);

% calculate normal force and sideforce
P_N_y = -C_N_y*0.5*rho*Vaer_bezwzgl^2*S;
P_N_z = -C_N_z*0.5*rho*Vaer_bezwzgl^2*S;

R = [P_x_x; P_N_y; P_N_z];
